simulink model "OL_BMO"  (R2024b)
settings: Solver=FixedStepDiscrete  StartTime=0.0  StopTime=final_time  FixedStep=0.1  RelTol=1e-3  EnableMultiTasking=on
settings Model: Creator=nctzv8  LastModifiedBy=voillat
settings ConfigSet: Description=OpenECU configuration set for code generation under RTW-EC.
settings SolverCC: AlgebraicLoopSolver=TrustRegion  PositivePriorityOrder=on
settings DataIOCC: LimitDataPoints=on  SaveFormat=Array  SignalLoggingSaveFormat=ModelDataLogs
settings OptimizationCC: DefaultParameterBehavior=Inlined  InlineInvariantSignals=on  ExpressionDepthLimit=2147483647  StateBitsets=on  DataBitsets=on  ZeroExternalMemoryAtStartup=off  ZeroInternalMemoryAtStartup=off  NoFixptDivByZeroProtection=on  EfficientFloat2IntCast=on  LifeSpan=1  EfficientTunableParamExpr=on
settings DebuggingCC: SaveWithParameterizedLinksMsg=none  SignalResolutionControl=TryResolveAllWithWarning  MultiTaskDSMMsg=warning  MultiTaskCondExecSysMsg=none  SingleTaskRateTransMsg=error  CheckMatrixSingularityMsg=warning  VectorMatrixConversionMsg=warning  SignalLabelMismatchMsg=warning  UnconnectedInputMsg=warning  UnconnectedOutputMsg=warning  UnconnectedLineMsg=warning  AllowSymbolicDim=off  StateNameClashWarn=warning  SFUnexpectedBacktrackingDiag=warning  SFNoUnconditionalDefaultTransitionDiag=warning  SFExecutionAtInitializationDiag=none  ArithmeticOperatorsInVariantConditions=warning
settings HardwareCC: ProdBitPerPointer=32  ProdBitPerSizeT=32  ProdBitPerPtrDiffT=32  ProdLargestAtomicInteger=Long  ProdLargestAtomicFloat=Double  ProdEndianess=BigEndian  ProdWordSize=32  ProdHWDeviceType=Freescale->32-bit PowerPC  TargetIntDivRoundTo=Zero  TargetEndianess=BigEndian  TargetHWDeviceType=Freescale->32-bit PowerPC  ProdEqTarget=off
settings ModelReferenceCC: EnableRefExpFcnMdlSchedulingChecks=on  PropagateSignalLabelsOutOfModel=off
settings SFSimCC: SimUseLocalCustomCode=off  MATLABDynamicMemAlloc=off  CustomCodeUndefinedFunction=UseInterfaceOnly
settings RTWCC: Description=OpenECU Platform Target (ERT, optimised floating-point code)  SystemTargetFile=openecu_ert.tlc  MakeCommand=make_rtw optimized_floating_point=1  TemplateMakefile=openecu_ert_r2015b_64.tmf  RetainRTWFile=on  RTWUseLocalCustomCode=off  IncludeHyperlinkInReport=on  GPUComputeCapability=3.5
settings CodeAppCC: ForceParamTrailComments=on  IgnoreCustomStorageClasses=off  SimulinkDataObjDesc=on  CustomSymbolStrType=$N$R$M  InsertBlockDesc=on  StateflowObjectComments=on  InternalIdentifier=Classic
settings STFCustomTargetCC: TargetLibSuffix=.a  GenerateSampleERTMain=on  IncludeMdlTerminateFcn=off  CombineOutputUpdateFcns=on  IncludeFileDelimiter=UseQuote  ERTCustomFileBanners=on  SupportContinuousTime=off  RemoveResetFunc=on  MATLABClassNameForMDSCustomization=Simulink.SoftwareTarget.ERTCustomization  SystemTargetFile=openecu_ert.tlc
settings ERTTargetCC: MultiwordLength=2048  GenerateSampleERTMain=on  ParMdlRefBuildCompliant=off  CompOptLevelCompliant=off  ConcurrentExecutionCompliant=off  IncludeMdlTerminateFcn=off  IncludeFileDelimiter=UseQuote  SupportNonInlinedSFcns=on  ModelStepFunctionPrototypeControlCompliant=off  CPPClassGenCompliant=off  UseToolchainInfoCompliant=off  ExtModeMexFile=noextcomm  ERTSrcFileBannerTemplate=oe_code_c_template.cgt  ERTHdrFileBannerTemplate=oe_code_h_template.cgt  ERTDataSrcFileTemplate=oe_data_c_template.cgt  ERTDataHdrFileTemplate=oe_data_h_template.cgt  ERTCustomFileTemplate=example_file_process.tlc  GlobalDataDefinition=InSeparateSourceFile  GlobalDataReference=InSeparateHeaderFile  ConvertIfToSwitch=off  SuppressUnreachableDefaultCases=off  EnableUserReplacementTypes=on  DynamicArrayContainerType=coder::array
settings ConfigComp: CovMetricSettings=dw  CovSaveCumulativeToWorkspaceVar=on  CovSaveSingleToWorkspaceVar=on  CovExternalEMLEnable=off

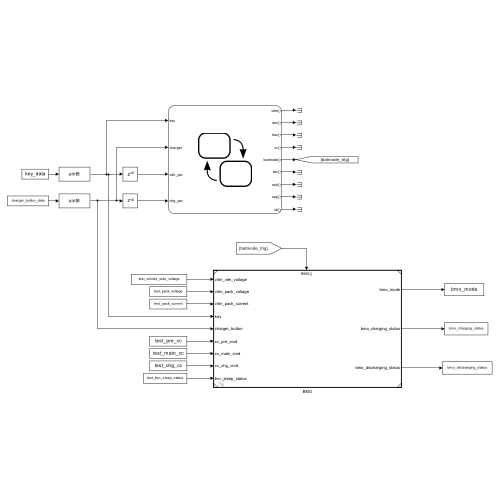
[thumbnail: Simulink's stored preview of the top-level diagram]
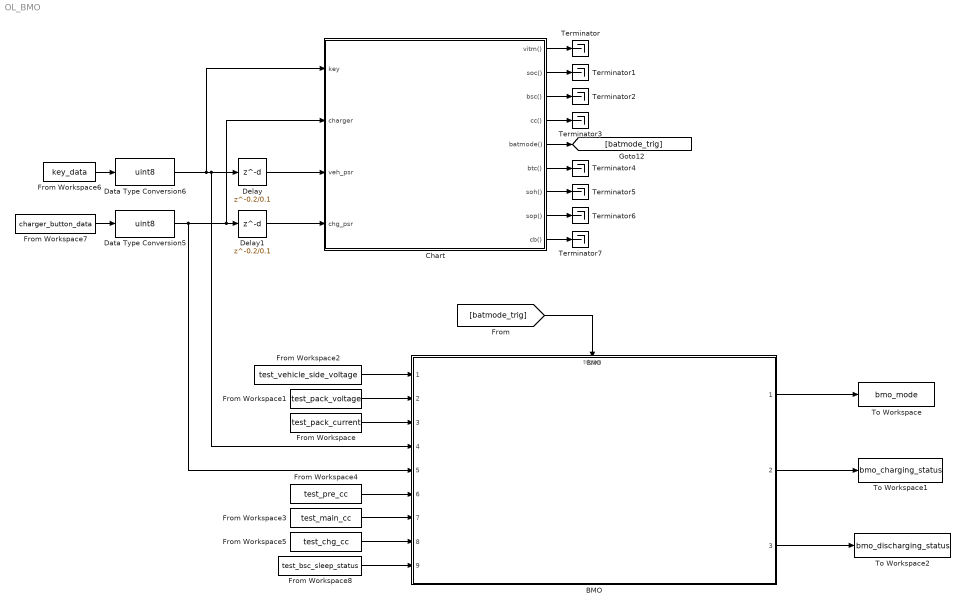
== system OL_BMO ==
  BMO : ModelReference  ModelNameDialog=BMO.slx  SimulationMode=Normal  ModelReferenceVersion=15.2  TriggerPortName=Trigger  TriggerPortTriggerType=function-call  TriggerPortStatesWhenEnabling=held
  Chart : Stateflow chart  TreatAsAtomicUnit=on
  Data Type Conversion5 : DataTypeConversion  OutDataTypeStr=uint8  SaturateOnIntegerOverflow=off  RndMeth=Floor
  Data Type Conversion6 : DataTypeConversion  OutDataTypeStr=uint8  SaturateOnIntegerOverflow=off  RndMeth=Floor
  Delay : Delay  DelayLength=0.2/0.1
  Delay1 : Delay  DelayLength=0.2/0.1
  From Workspace : FromWorkspace  VariableName=test_pack_current  SampleTime=-1
  From Workspace1 : FromWorkspace  VariableName=test_pack_voltage  SampleTime=-1
  From Workspace2 : FromWorkspace  VariableName=test_vehicle_side_voltage  SampleTime=-1
  From Workspace3 : FromWorkspace  VariableName=test_main_cc  SampleTime=-1
  From Workspace4 : FromWorkspace  VariableName=test_pre_cc  SampleTime=-1
  From Workspace5 : FromWorkspace  VariableName=test_chg_cc  SampleTime=-1
  From Workspace6 : FromWorkspace  VariableName=key_data  SampleTime=-1
  From Workspace7 : FromWorkspace  VariableName=charger_button_data  SampleTime=-1
  From Workspace8 : FromWorkspace  VariableName=test_bsc_sleep_status  SampleTime=-1
  Terminator{,1..7} (8 alike) : Terminator
  To Workspace : ToWorkspace  VariableName=bmo_mode  SaveFormat=Timeseries  SampleTime=-1
  To Workspace1 : ToWorkspace  VariableName=bmo_charging_status  SaveFormat=Timeseries  SampleTime=-1
  To Workspace2 : ToWorkspace  VariableName=bmo_discharging_status  SaveFormat=Timeseries  SampleTime=-1
  wires:
  BMO/1 -> To Workspace/1
  BMO/2 -> To Workspace1/1
  BMO/3 -> To Workspace2/1
  [batmode_trig] -> BMO/Trigger
  Chart/1(vitm()) -> Terminator/1
  Chart/2(soc()) -> Terminator1/1
  Chart/3(bsc()) -> Terminator2/1
  Chart/4(cc()) -> Terminator3/1
  Chart/5(batmode()) -> [batmode_trig]
  Chart/6(btc()) -> Terminator4/1
  Delay/1 -> Chart/3(veh_psr)
  Chart/7(soh()) -> Terminator5/1
  Chart/8(sop()) -> Terminator6/1
  Chart/9(cb()) -> Terminator7/1
  Delay1/1 -> Chart/4(chg_psr)
  Data Type Conversion5/1 -> BMO/5, Chart/2(charger), Delay1/1
  Data Type Conversion6/1 -> Chart/1(key), BMO/4, Delay/1
  From Workspace6/1 -> Data Type Conversion6/1
  From Workspace7/1 -> Data Type Conversion5/1
  From Workspace/1 -> BMO/3
  From Workspace1/1 -> BMO/2
  From Workspace2/1 -> BMO/1
  From Workspace3/1 -> BMO/7
  From Workspace4/1 -> BMO/6
  From Workspace5/1 -> BMO/8
  From Workspace8/1 -> BMO/9

== stateflow chart OL_BMO/Chart ==
  state main_chg
    (default) -> (junction 607)
    main_chg -> (junction 607) [order 1]
    (junction 607) -> (junction 606) : {vitm;}
    (junction 606) -> (junction 597) : {soc;}
    (junction 597) -> (junction 612) : {bsc;}
    (junction 612) -> (junction 598) : {soh;}
    (junction 598) -> (junction 604) : {cc;}
    (junction 604) -> (junction 605) : {batmode;}
    (junction 605) -> (junction 592) : {btc;}
    (junction 592) -> (junction 593) : {sop;}
    (junction 593) -> (junction 594) : {cb;}
  state main_key
    (default) -> (junction 544)
    main_key -> (junction 544) [order 1]
    (junction 544) -> (junction 543) : {vitm;}
    (junction 543) -> (junction 534) : {soc;}
    (junction 534) -> (junction 549) : {bsc;}
    (junction 549) -> (junction 535) : {soh;}
    (junction 535) -> (junction 541) : {cc;}
    (junction 541) -> (junction 542) : {batmode;}
    (junction 542) -> (junction 529) : {btc;}
    (junction 529) -> (junction 530) : {sop;}
    (junction 530) -> (junction 531) : {cb;}
  state init_key
    (default) -> (junction 81)
    init_key -> (junction 81) [order 1]
    (junction 81) -> (junction 83) : {vitm;}
    (junction 83) -> (junction 89) : {soc;}
    (junction 89) -> (junction 527) : {bsc;}
    (junction 527) -> (junction 82) : {soh;}
    (junction 82) -> (junction 85) : {cc;}
    (junction 85) -> (junction 87) : {batmode;}
    (junction 87) -> (junction 158) : {btc;}
    (junction 158) -> (junction 195) : {sop;}
    (junction 195) -> (junction 236) : {cb;}
  state init_chg
    (default) -> (junction 586)
    init_chg -> (junction 586) [order 1]
    (junction 586) -> (junction 585) : {vitm;}
    (junction 585) -> (junction 576) : {soc;}
    (junction 576) -> (junction 591) : {bsc;}
    (junction 591) -> (junction 577) : {soh;}
    (junction 577) -> (junction 583) : {cc;}
    (junction 583) -> (junction 584) : {batmode;}
    (junction 584) -> (junction 571) : {btc;}
    (junction 571) -> (junction 572) : {sop;}
    (junction 572) -> (junction 573) : {cb;}
  state no_power
    entry:
    end_count =0;
  state end_key
    exit:
    end_count = end_count +1;
    (default) -> (junction 565)
    end_key -> (junction 565) [order 1]
    (junction 565) -> (junction 564) : {vitm;}
    (junction 564) -> (junction 555) : {soc;}
    (junction 555) -> (junction 570) : {bsc;}
    (junction 570) -> (junction 556) : {soh;}
    (junction 556) -> (junction 562) : {cc;}
    (junction 562) -> (junction 563) : {batmode;}
    (junction 563) -> (junction 550) : {btc;}
    (junction 550) -> (junction 551) : {sop;}
    (junction 551) -> (junction 552) : {cb;}
  state end_chg
    exit:
    end_count = end_count +1;
    (default) -> (junction 628)
    end_chg -> (junction 628) [order 1]
    (junction 628) -> (junction 627) : {vitm;}
    (junction 627) -> (junction 618) : {soc;}
    (junction 618) -> (junction 633) : {bsc;}
    (junction 633) -> (junction 619) : {soh;}
    (junction 619) -> (junction 625) : {cc;}
    (junction 625) -> (junction 626) : {batmode;}
    (junction 626) -> (junction 613) : {btc;}
    (junction 613) -> (junction 614) : {sop;}
    (junction 614) -> (junction 615) : {cb;}
  (default) -> no_power
  no_power -> init_chg [order 2] : [charger > 0.5]
  no_power -> init_key [order 1] : [key > 0.5]
  end_chg -> no_power [order 2]
  end_key -> no_power [order 2]
  init_key -> main_key [order 1]
  init_chg -> main_chg [order 1]
  main_chg -> end_chg [order 1] : [chg_psr < 0.5]
  main_key -> end_key [order 1] : [veh_psr < 0.5]
  end_key -> end_key [order 1] : [end_count < 10]
  end_chg -> end_chg [order 1] : [end_count < 10]
  data: key input; charger input; veh_psr input; end_count local double =0; chg_psr input
  events: vitm output FUNCTION_CALL_EVENT; soc output FUNCTION_CALL_EVENT; bsc output FUNCTION_CALL_EVENT; cc output FUNCTION_CALL_EVENT; batmode output FUNCTION_CALL_EVENT; btc output FUNCTION_CALL_EVENT; soh output FUNCTION_CALL_EVENT; sop output FUNCTION_CALL_EVENT; cb output FUNCTION_CALL_EVENT
